simulink model "fig1_26_simulink"  (R2021b)
settings: Solver=ode45  StartTime=0.0  StopTime=44  RelTol=1e-3  EnableMultiTasking=on
model workspace (MAT data in the model file):
  X0 = 0
values from neighbouring files (symbols this model uses):
  b = 8/3    (= 2.66666666667)    [fig1_27.m]    (also in fig1_28.m; fig1_29.m; fig1_30.m; fig1_32.m)
  p = 10    [fig1_27.m]    (also in fig1_28.m; fig1_29.m; fig1_30.m; fig1_32.m)
  r = 0.5    [fig1_27.m]    (also in fig1_28.m = 2; fig1_29.m = 25; fig1_30.m = 160; fig1_32.m = 143)
settings Model: Creator=One Informatic  LastModifiedBy=One Informatic
settings DataIOCC: LimitDataPoints=on  SaveFormat=Array  SignalLoggingSaveFormat=ModelDataLogs  ReturnWorkspaceOutputs=off  SignalLoggingName=sigsOut
settings DebuggingCC: SaveWithParameterizedLinksMsg=none  UnderspecifiedInitializationDetection=Classic  MergeDetectMultiDrivingBlocksExec=none  SignalResolutionControl=TryResolveAllWithWarning  MultiTaskDSMMsg=warning  MultiTaskCondExecSysMsg=none
settings HardwareCC: ProdBitPerPointer=32  ProdBitPerSizeT=32  ProdBitPerPtrDiffT=32  ProdLargestAtomicFloat=None  ProdIntDivRoundTo=Undefined  ProdEndianess=Unspecified  ProdWordSize=32  ProdHWDeviceType=32-bit Generic  TargetUnknown=on
settings ModelReferenceCC: PropagateSignalLabelsOutOfModel=off
settings GRTTargetCC: CombineOutputUpdateFcns=off  GRTInterface=on
settings ConfigComp: CovMetricSettings=dw  CovSaveCumulativeToWorkspaceVar=on  CovSaveSingleToWorkspaceVar=on

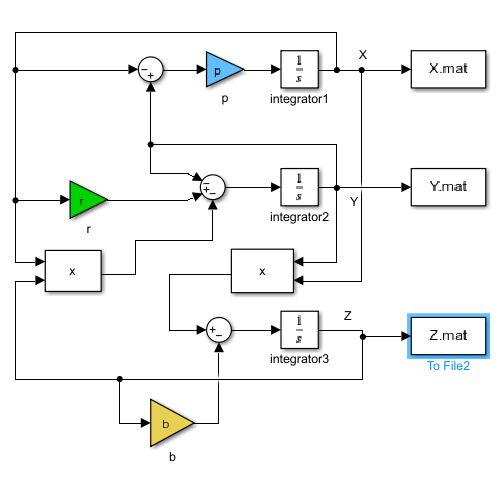
[thumbnail: Simulink's stored preview of the top-level diagram]
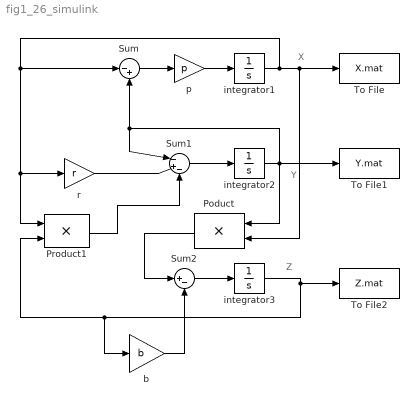
== system fig1_26_simulink ==
  note: X
  note: Y
  note: Z
  Poduct : Product  SaturateOnIntegerOverflow=on  OutDataTypeStr=Inherit: Same as first input
  Product1 : Product  SaturateOnIntegerOverflow=on  OutDataTypeStr=Inherit: Same as first input
  Sum : Sum  Inputs=|-+  SaturateOnIntegerOverflow=on
  Sum1 : Sum  Inputs=|-+-  SaturateOnIntegerOverflow=on
  Sum2 : Sum  Inputs=|+-  SaturateOnIntegerOverflow=on
  To File : ToFile  Filename=X.mat  MatrixName=X  SampleTime=0.001
  To File1 : ToFile  Filename=Y.mat  MatrixName=Y  SampleTime=0.001
  To File2 : ToFile  Filename=Z.mat  MatrixName=Z  SampleTime=0.001
  b : Gain  Gain=b  SaturateOnIntegerOverflow=on  OutDataTypeStr=Inherit: Same as input  ParamDataTypeStr=Inherit: Same as input
  integrator1 : Integrator  InitialCondition=20
  integrator2 : Integrator  InitialCondition=166
  integrator3 : Integrator  InitialCondition=163
  p : Gain  Gain=p  SaturateOnIntegerOverflow=on  OutDataTypeStr=Inherit: Same as input  ParamDataTypeStr=Inherit: Same as input
  r : Gain  Gain=r  SaturateOnIntegerOverflow=on  OutDataTypeStr=Inherit: Same as input  ParamDataTypeStr=Inherit: Same as input
  wires:
  Sum2/1 -> integrator3/1
  Sum1/1 -> integrator2/1
  integrator1/1 -> Poduct/2, To File/1, r/1, Product1/1, Sum/1
  integrator2/1 -> To File1/1, Sum1/1, Sum/2, Poduct/1
  r/1 -> Sum1/2
  Product1/1 -> Sum1/3
  integrator3/1 -> To File2/1, Product1/2, b/1
  b/1 -> Sum2/2
  Poduct/1 -> Sum2/1
  Sum/1 -> p/1
  p/1 -> integrator1/1
